simulink model "Encoder"  (R2018b)
settings: Solver=FixedStepAuto  StartTime=0.0  StopTime=inf  RelTol=1e-3
settings Model: SimulationMode=external  ExtModeTrigDuration=2  Creator=lbai  LastModifiedBy=lbai
settings OptimizationCC: EnhancedBackFolding=on  PassReuseOutputArgsAs=Individual arguments  MaxStackSize=64  OptimizeBlockOrder=speed  DifferentSizesBufferReuse=on  OptimizationCustomize=off
settings DebuggingCC: ParameterTunabilityLossMsg=error
settings HardwareCC: ProdBitPerInt=16  ProdBitPerPointer=16  ProdBitPerSizeT=16  ProdBitPerPtrDiffT=16  ProdLargestAtomicFloat=None  ProdWordSize=8  ProdHWDeviceType=Atmel->AVR
settings SFSimCC: MATLABDynamicMemAlloc=off
settings RTWCC: SystemTargetFile=ert.tlc  HardwareBoard=Arduino Mega 2560  TemplateMakefile=ert_default_tmf  GenerateReport=on  Toolchain=Arduino AVR  BuildConfiguration=Faster Runs  IncludeHyperlinkInReport=on  LaunchReport=on  GenerateTraceInfo=on  GenerateTraceReport=on  GenerateTraceReportSl=on  GenerateTraceReportSf=on  GenerateTraceReportEml=on
settings CodeAppCC: ForceParamTrailComments=on  IgnoreCustomStorageClasses=off  OperatorAnnotations=on  SimulinkDataObjDesc=on  SFDataObjDesc=on  InsertBlockDesc=on
settings ERTTargetCC: SupportContinuousTime=on  SupportVariableSizeSignals=on

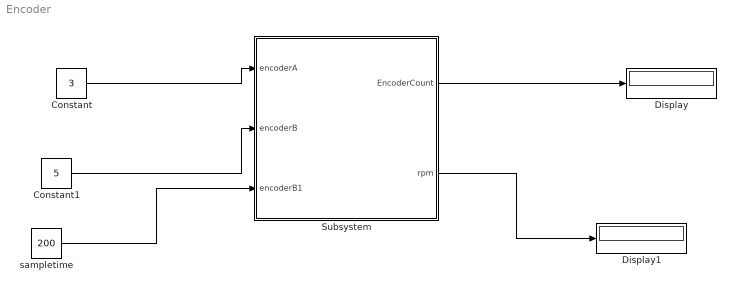
== system Encoder ==
  Constant : Constant  Value=3  OutDataTypeStr=uint8
  Constant1 : Constant  Value=5  OutDataTypeStr=uint8
  Display : Display
  Display1 : Display
  Subsystem : Subsystem
      mask Display:
      | image('halleffect.jpg');
      | port_label('input', 1, 'A')
      | port_label('input', 2, 'B')
      | port_label('input', 3, 'sampleTIME')
      | port_label('output', 1, 'counter')
      | port_label('output', 2, 'rpm')
  "sampletime " : Constant  Value=200  OutDataTypeStr=uint16
  wires:
  Constant/1 -> Subsystem/1(encoderA)
  Constant1/1 -> Subsystem/2(encoderB)
  Subsystem/1(EncoderCount) -> Display/1
  Subsystem/2("rpm ") -> Display1/1
  "sampletime "/1 -> Subsystem/3(encoderB1)

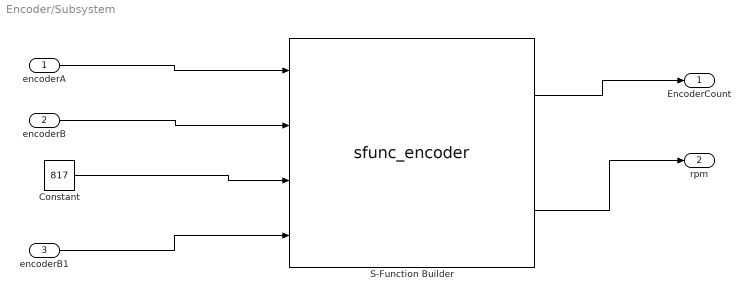
== system Encoder/Subsystem ==
  encoderA : Inport
  encoderB : Inport  Port=2
  encoderB1 : Inport  Port=3
  Constant : Constant  Value=817  OutDataTypeStr=uint32
  S-Function Builder : S-Function  InitFcn=try, set_param(gcb,'FunctionName','sfunc_encoder'), end  FunctionName=sfunc_encoder  SFunctionModules=sfunc_encoder_wrapper  SFunctionDeploymentMode=off  EnableBusSupport=off  mask(S-Function Builder){}
      mask help: Simulink:masks:SFunctionBuilder_MD
      mask init:
      | val = [[.9  0.75 0.75 1 1 .9 .9 1]',[1 1 0.75 0.75 .9 .9 1 .9]'];try , sys = get_param(gcb,'SfunBuilderFcnName');if isempty(sys), sys = get_param(gcb,'FunctionName'); end,catch, sys = get_param(gcb,'FunctionName'); end
      settings: CopyFcn=set_param(gcbh,'LinkStatus','none')  PreSaveFcn=try, set_param(gcb,'FunctionName','sfunc_encoder'), end  OpenFcn=sfunctionwizard(gcbh)
      mask Display: plot(val(:,1),val(:,2)),disp(sys), port_label('input',1,'pinA'), port_label('input',2,'pinB'), port_label('input',3,'cntperrot'), port_label('input',4,'sampletime'), port_label('output',1,'pos'), port_label('output',2,'rpm')
  EncoderCount : Outport
  "rpm " : Outport  Port=2
  wires:
  encoderB/1 -> S-Function Builder/2
  encoderA/1 -> S-Function Builder/1
  S-Function Builder/1 -> EncoderCount/1
  S-Function Builder/2 -> "rpm "/1
  Constant/1 -> S-Function Builder/3
  encoderB1/1 -> S-Function Builder/4
